simulink library "M160_lib"  (Simulink 7.8)
settings: Solver=FixedStepDiscrete  StartTime=0.0  StopTime=10.0  RelTol=1e-3
PreLoadFcn:
  | update_path
undefined symbols (not defined in the file): Afr_atCool2facLambdaReqCorr_CUR_x, Afr_atCool2facLambdaReqCorr_CUR_y, Afr_atMani2facLambdaReqCorr_CUR_x, Afr_atMani2facLambdaReqCorr_CUR_y, Afr_facLambdaReqMan, Afr_facRatioMan, Afr_facStoich, Afr_flgLambdaReqOverride, Afr_flgRatioOverride, Afr_rpmEngSpdfacRelAir2facLambdaReqBase_MAP_x, Afr_rpmEngSpdfacRelAir2facLambdaReqBase_MAP_y, Afr_rpmEngSpdfacRelAir2facLambdaReqBase_MAP_z, Ais_flgAirInjReacPumpOverride, Ais_stAirInjReacPumpMan, Amc_flgAirMassFlowOverride, Amc_uSens2AirMassFlow_CUR_x, Amc_uSens2AirMassFlow_CUR_y, Amc_uSensMaxValid, Amc_uSensMinValid, Amf_facRelAirMan, Amf_flgAirMassPerStrOverride, Amf_flgRelAirOverride, Amf_flgSwitch2AirMassFlowMeter, Amf_mAirPerStrMan, Amf_pManiEngSpd2facRelAirCorr_MAP_x, Amf_pManiEngSpd2facRelAirCorr_MAP_y, Amf_pManiEngSpd2facRelAirCorr_MAP_z, Amf_rpmEngSpd2facTempCorr_CUR_x, Amf_rpmEngSpd2facTempCorr_CUR_y, Amf_shcSpecGasConst_C, Amf_volEngDisp_C, Apv_facAirPumpRateMan, Apv_factor, Apv_flgAirPumpRateOverride, Apv_tiPeriod_C, Bvc_rVoltDivHigh, Bvc_rVoltDivLow, Bvc_uBattMax, Bvc_uBattMin, CDRV_E_OK_, Cov_facChOverVlvRateMan, Cov_factor, Cov_flgChOverVlvRateOverride, Cov_tiPeriod_C, Cpc_atManiTmp2facPresCorr_CUR_x, Cpc_atManiTmp2facPresCorr_CUR_y, Cpc_flgPChargeOverride, Cpc_uSens2pManiBase_CUR_x, Cpc_uSens2pManiBase_CUR_y, Ctc_rPullUp_C, Ctc_rSens2atCool_CUR_x, Ctc_rSens2atCool_CUR_y, Ctc_uSensMaxValid, Ctc_uSensMinValid, Ctc_uSupply, Doh_OutputDiagnosisOverride, dummy_facAirPumpRateReq, dummy_facChOverVlvRateReq, dummy_flgInterCoolerOverride, dummy_flgKl50Override ... (+243)
libraries: simulink x36, ehooks_lib x3
(part 8 of 8)

== system M160_lib/Sensors/Cpc/Cpc_get/G1_ADC_Input_Receive ==
  Data Type Conversion2 : DataTypeConversion  OutMin=0.0  OutMax=5.0  OutDataTypeStr=single
  Data Type Conversion3 : DataTypeConversion  OutMin=0.0  OutMax=1.0  OutDataTypeStr=boolean
  FlexECU_DevLib_FcnAPI_Wrapper_SFcn : S-Function  FunctionName=ehooks_medc17flex_devlib_basic_io_fcncall  Parameters=NoInputPorts, NoOutputPorts, InputPortDataTypes, OutputPortDataTypes, CFunctionArgTypes, CFunctionName, ChannelName  EnableBusSupport=off  mask{NoInputPorts=0, NoOutputPorts=2, InputPortDataTypes=, OutputPortDataTypes=uint8,int16, CFunctionArgTypes=ret,ref, CFunctionName=DevLib_Adc_Get, ChannelName=I_A_AN05}
      mask prompts: NoInputPorts "Number of input ports"; NoOutputPorts "Number of output ports"; InputPortDataTypes "Input port data types"; OutputPortDataTypes "Output port data types"; CFunctionArgTypes "C function argument types"; CFunctionName "C function name"; ChannelName "Channel (pin) name"
      mask Display: disp('EHOOKS FlexECU\nDevLib Wrapper\nS-Function')
  Gain : Gain  Gain=5/1023  OutDataTypeStr=Inherit: Same as input
  status : Outport
  uRaw : Outport  Port=2
  wires:
  FlexECU_DevLib_FcnAPI_Wrapper_SFcn/1 -> Data Type Conversion3/1
  FlexECU_DevLib_FcnAPI_Wrapper_SFcn/2 -> Data Type Conversion2/1
  Gain/1 -> uRaw/1
  Data Type Conversion3/1 -> status/1
  Data Type Conversion2/1 -> Gain/1

== system M160_lib/Sensors/Cpc/Cpc_pCharge_calc/ECU_FcnCallTrigger_Source_DownStream ==
  ECU_FcnCallTrigger_Source_SFcn : S-Function  Tag=ECU_FcnCallTrigger_Source_SFcn  Description=Internal S-function for custom block ECU_FcnCallTrigger_Source. Do not rename!  FunctionName=ehooks_fcncalltrigger_source  Parameters=FunctionBlockId, FunctionCName, ProcessName, TaskPeriod, TaskPriority  EnableBusSupport=off  mask(ECU_FcnCallTrigger_Source_SFcn){FunctionCName=Cpc_pCharge_calc, FunctionBlockId=SmartM160/Sensors/Cpc/Cpc_pCharge_calc, ProcessName=BypEasyhooks_S0_Pre_Proc, TaskPriority=0, TaskPeriod=1}
      mask prompts: FunctionCName "Function C name"; FunctionBlockId "Function block identifier"; ProcessName "Process name"; TaskPriority "Task priority (0..255)"; TaskPeriod "Sample time (0 for asynchronous operation)"
      mask help: Internal S-function for custom block ECU_FcnCallTrigger_Source. Do not rename!
      mask Display: disp('EHOOKS ECU Trigger\nSource S-Function')
  TriggerOut : Outport
  wires:
  ECU_FcnCallTrigger_Source_SFcn/1 -> TriggerOut/1

== system M160_lib/Sensors/Cpc/Cpc_pCharge_get/ECU_FcnCallTrigger_Source_DownStream ==
  ECU_FcnCallTrigger_Source_SFcn : S-Function  Tag=ECU_FcnCallTrigger_Source_SFcn  Description=Internal S-function for custom block ECU_FcnCallTrigger_Source. Do not rename!  FunctionName=ehooks_fcncalltrigger_source  Parameters=FunctionBlockId, FunctionCName, ProcessName, TaskPeriod, TaskPriority  EnableBusSupport=off  mask(ECU_FcnCallTrigger_Source_SFcn){FunctionCName=Cpc_pCharge_get, FunctionBlockId=SmartM160/Sensors/Cpc/Cpc_pCharge_get, ProcessName=BypEasyhooks_1ms_Pre_Proc, TaskPriority=0, TaskPeriod=1}
      mask prompts: FunctionCName "Function C name"; FunctionBlockId "Function block identifier"; ProcessName "Process name"; TaskPriority "Task priority (0..255)"; TaskPeriod "Sample time (0 for asynchronous operation)"
      mask help: Internal S-function for custom block ECU_FcnCallTrigger_Source. Do not rename!
      mask Display: disp('EHOOKS ECU Trigger\nSource S-Function')
  TriggerOut : Outport
  wires:
  ECU_FcnCallTrigger_Source_SFcn/1 -> TriggerOut/1

== system M160_lib/Sensors/Mpc/Mpc_calc/Accumulator ==
  in : Inport
  initValue : Inport  Port=2
  Add : Sum
  MATLAB Function : MATLAB Function  TreatAsAtomicUnit=on
  Switch2 : Switch  Threshold=1
  Unit Delay : UnitDelay  SampleTime=-1
  Out2 : Outport
  wires:
  MATLAB Function/1(y) -> Switch2/2
  Add/1 -> Unit Delay/1, Switch2/1
  initValue/1 -> Switch2/3
  Switch2/1 -> Out2/1
  Unit Delay/1 -> Add/2
  in/1 -> MATLAB Function/1(u), Add/1

== system M160_lib/Sensors/Mpc/Mpc_calc/Counter ==
  in : Inport
  Add1 : Sum
  Constant1 : Constant  OutDataTypeStr=single
  Constant2 : Constant  Value=0  OutDataTypeStr=single
  MATLAB Function : MATLAB Function  TreatAsAtomicUnit=on
  Switch2 : Switch  Threshold=1
  Unit Delay1 : UnitDelay  SampleTime=-1
  Out1 : Outport
  wires:
  in/1 -> MATLAB Function/1(u)
  MATLAB Function/1(y) -> Switch2/2
  Add1/1 -> Unit Delay1/1, Switch2/1
  Constant2/1 -> Switch2/3
  Switch2/1 -> Out1/1
  Unit Delay1/1 -> Add1/2
  Constant1/1 -> Add1/1

== system M160_lib/Sensors/Mpc/Mpc_get/G1_ADC_Input_Receive ==
  Data Type Conversion2 : DataTypeConversion  OutMin=0.0  OutMax=5.0  OutDataTypeStr=single
  Data Type Conversion3 : DataTypeConversion  OutMin=0.0  OutMax=1.0  OutDataTypeStr=boolean
  FlexECU_DevLib_FcnAPI_Wrapper_SFcn : S-Function  FunctionName=ehooks_medc17flex_devlib_basic_io_fcncall  Parameters=NoInputPorts, NoOutputPorts, InputPortDataTypes, OutputPortDataTypes, CFunctionArgTypes, CFunctionName, ChannelName  EnableBusSupport=off  mask{NoInputPorts=0, NoOutputPorts=2, InputPortDataTypes=, OutputPortDataTypes=uint8,int16, CFunctionArgTypes=ret,ref, CFunctionName=DevLib_Adc_Get, ChannelName=I_A_AN05}
      mask prompts: NoInputPorts "Number of input ports"; NoOutputPorts "Number of output ports"; InputPortDataTypes "Input port data types"; OutputPortDataTypes "Output port data types"; CFunctionArgTypes "C function argument types"; CFunctionName "C function name"; ChannelName "Channel (pin) name"
      mask Display: disp('EHOOKS FlexECU\nDevLib Wrapper\nS-Function')
  Gain : Gain  Gain=5/1023  OutDataTypeStr=Inherit: Same as input
  status : Outport
  uRaw : Outport  Port=2
  wires:
  Data Type Conversion2/1 -> Gain/1
  Data Type Conversion3/1 -> status/1
  Gain/1 -> uRaw/1
  FlexECU_DevLib_FcnAPI_Wrapper_SFcn/2 -> Data Type Conversion2/1
  FlexECU_DevLib_FcnAPI_Wrapper_SFcn/1 -> Data Type Conversion3/1

== system M160_lib/Sensors/Mpc/Mpc_pMani_calc/ECU_FcnCallTrigger_Source_DownStream ==
  ECU_FcnCallTrigger_Source_SFcn : S-Function  Tag=ECU_FcnCallTrigger_Source_SFcn  Description=Internal S-function for custom block ECU_FcnCallTrigger_Source. Do not rename!  FunctionName=ehooks_fcncalltrigger_source  Parameters=FunctionBlockId, FunctionCName, ProcessName, TaskPeriod, TaskPriority  EnableBusSupport=off  mask(ECU_FcnCallTrigger_Source_SFcn){FunctionCName=Mpc_pMani_calc, FunctionBlockId=SmartM160/Sensors/Mpc/Mpc_pMani_calc, ProcessName=BypEasyhooks_S0_Pre_Proc, TaskPriority=0, TaskPeriod=1}
      mask prompts: FunctionCName "Function C name"; FunctionBlockId "Function block identifier"; ProcessName "Process name"; TaskPriority "Task priority (0..255)"; TaskPeriod "Sample time (0 for asynchronous operation)"
      mask help: Internal S-function for custom block ECU_FcnCallTrigger_Source. Do not rename!
      mask Display: disp('EHOOKS ECU Trigger\nSource S-Function')
  TriggerOut : Outport
  wires:
  ECU_FcnCallTrigger_Source_SFcn/1 -> TriggerOut/1

== system M160_lib/Sensors/Mpc/Mpc_pMani_get/ECU_FcnCallTrigger_Source_DownStream ==
  ECU_FcnCallTrigger_Source_SFcn : S-Function  Tag=ECU_FcnCallTrigger_Source_SFcn  Description=Internal S-function for custom block ECU_FcnCallTrigger_Source. Do not rename!  FunctionName=ehooks_fcncalltrigger_source  Parameters=FunctionBlockId, FunctionCName, ProcessName, TaskPeriod, TaskPriority  EnableBusSupport=off  mask(ECU_FcnCallTrigger_Source_SFcn){FunctionCName=Mpc_pMani_get, FunctionBlockId=SmartM160/Sensors/Mpc/Mpc_pMani_get, ProcessName=BypEasyhooks_1ms_Pre_Proc, TaskPriority=0, TaskPeriod=1}
      mask prompts: FunctionCName "Function C name"; FunctionBlockId "Function block identifier"; ProcessName "Process name"; TaskPriority "Task priority (0..255)"; TaskPeriod "Sample time (0 for asynchronous operation)"
      mask help: Internal S-function for custom block ECU_FcnCallTrigger_Source. Do not rename!
      mask Display: disp('EHOOKS ECU Trigger\nSource S-Function')
  TriggerOut : Outport
  wires:
  ECU_FcnCallTrigger_Source_SFcn/1 -> TriggerOut/1

== system M160_lib/Actuators/Tvc/ThrottleValveControl/PID_Limit_AWU/Limiter ==
  max : Inport
  in : Inport  Port=2
  min : Inport  Port=3
  Saturation Dynamic : simulink/Discontinuities/Saturation Dynamic  OutMin=[]  OutMax=[]  OutDataTypeStr=Inherit: Same as second input  OutDataType=fixdt(1, 16)  OutScaling=2^-10  DoSatur=off
  return : Outport
  wires:
  max/1 -> Saturation Dynamic/1
  in/1 -> Saturation Dynamic/2
  min/1 -> Saturation Dynamic/3
  Saturation Dynamic/1 -> return/1

== system M160_lib/Functions/Lcc/PID-Controller/PID_Limit_AWU/Limiter ==
  max : Inport
  in : Inport  Port=2
  min : Inport  Port=3
  Saturation Dynamic : simulink/Discontinuities/Saturation Dynamic  OutMin=[]  OutMax=[]  OutDataTypeStr=Inherit: Same as second input  OutDataType=fixdt(1, 16)  OutScaling=2^-10  DoSatur=off
  return : Outport
  wires:
  max/1 -> Saturation Dynamic/1
  in/1 -> Saturation Dynamic/2
  min/1 -> Saturation Dynamic/3
  Saturation Dynamic/1 -> return/1

== system M160_lib/Functions/T2t/ThrottleValveControl/PID_Limit_AWU/Limiter ==
  max : Inport
  in : Inport  Port=2
  min : Inport  Port=3
  Saturation Dynamic : simulink/Discontinuities/Saturation Dynamic  OutMin=[]  OutMax=[]  OutDataTypeStr=Inherit: Same as second input  OutDataType=fixdt(1, 16)  OutScaling=2^-10  DoSatur=off
  return : Outport
  wires:
  max/1 -> Saturation Dynamic/1
  in/1 -> Saturation Dynamic/2
  min/1 -> Saturation Dynamic/3
  Saturation Dynamic/1 -> return/1

== system M160_lib/Functions/T2t/WastegateControl/PID_Limit_AWU/Limiter ==
  max : Inport
  in : Inport  Port=2
  min : Inport  Port=3
  Saturation Dynamic : simulink/Discontinuities/Saturation Dynamic  OutMin=[]  OutMax=[]  OutDataTypeStr=Inherit: Same as second input  OutDataType=fixdt(1, 16)  OutScaling=2^-10  DoSatur=off
  return : Outport
  wires:
  Saturation Dynamic/1 -> return/1
  min/1 -> Saturation Dynamic/3
  in/1 -> Saturation Dynamic/2
  max/1 -> Saturation Dynamic/1

== system M160_lib/Functions/Tqs/EngSpdControl/PID_Limit_AWU/Limiter ==
  max : Inport
  in : Inport  Port=2
  min : Inport  Port=3
  Saturation Dynamic : simulink/Discontinuities/Saturation Dynamic  OutMin=[]  OutMax=[]  OutDataTypeStr=Inherit: Same as second input  OutDataType=fixdt(1, 16)  OutScaling=2^-10  DoSatur=off
  return : Outport
  wires:
  max/1 -> Saturation Dynamic/1
  in/1 -> Saturation Dynamic/2
  min/1 -> Saturation Dynamic/3
  Saturation Dynamic/1 -> return/1

== matlab function Sensors/Egc/LowpassT/MATLAB Function ==
  data: x output double; u input double; y output double
function [x,y]= fcn(u)
% initValue Test
if(u<0)
    y = 0;
else
    y = 1;
end

x = u;

== matlab function Sensors/Egc/LowpassT_Fcn/MATLAB Function ==
  data: u input double; y output double
function y = fcn(u)
% initValue Test
if(u<0)
    y = 0;
else
    y = 1;
end

== matlab function Sensors/Cpc/Cpc_calc/Accumulator/MATLAB Function ==
  data: u input double; y output double
function y = fcn(u)
% initValue Test
if(u<=0)
    y = 0;
else
    y = 1;
end

== matlab function Sensors/Cpc/Cpc_calc/Counter/MATLAB Function ==
  data: u input double; y output double
function y = fcn(u)
% initValue Test
if(u<=0)
    y = 0;
else
    y = 1;
end

== matlab function Functions/Opm/OpMode/fcn_OpMode ==
  data: Opm_stEngControl input double; Opm_flgIOErrorAct input double; Opm_idxAct output double; Opm_flgIOErrorMemIn input double; Opm_flgIOErrorReset output double
function [Opm_idxAct,Opm_flgIOErrorReset]= fcn(Opm_stEngControl,Opm_flgIOErrorAct,Opm_flgIOErrorMemIn)
% fcn_OpMode

sm = single(0);
Opm_idxAct = single(0);
Opm_flgIOErrorReset = false;

if(sm==0)                                            % Off_state
        if(Opm_stEngControl)
            Opm_idxAct = single(1);
            sm = single(2);
        end
        if(Opm_flgIOErrorMemIn)
            Opm_idxAct = single(2);
            sm = single(1);
        end
        Opm_flgIOErrorReset = false;
end
if(sm==1)                                            % IOError_state
        if((~Opm_stEngControl)&&(~Opm_flgIOErrorAct))
            Opm_flgIOErrorReset = true;
            Opm_idxAct = single(0);
            sm = single(0);
        end
end
if(sm==2)                                            % Normal_state
        if(~Opm_stEngControl)
            Opm_idxAct = single(0);
            sm = single(0);
        end
        if(Opm_flgIOErrorMemIn)
            Opm_idxAct = single(2);
            sm = single(1);
        end
        Opm_flgIOErrorReset = false;
end

== matlab function Functions/Opm/ErrorCheck/Counter/MATLAB Function ==
  data: u input double; y output double
function y = fcn(u)
% initValue Test
if(u<=0)
    y = 0;
else
    y = 1;
end

== matlab function Functions/Opm/ErrorCheck/Counter1/MATLAB Function ==
  data: u input double; y output double
function y = fcn(u)
% initValue Test
if(u<=0)
    y = 0;
else
    y = 1;
end

== matlab function Functions/Opm/ErrorCheck/Counter2/MATLAB Function ==
  data: u input double; y output double
function y = fcn(u)
% initValue Test
if(u<=0)
    y = 0;
else
    y = 1;
end

== matlab function Sensors/Mpc/Mpc_calc/Accumulator/MATLAB Function ==
  data: u input double; y output double
function y = fcn(u)
% initValue Test
if(u<=0)
    y = 0;
else
    y = 1;
end

== matlab function Sensors/Mpc/Mpc_calc/Counter/MATLAB Function ==
  data: u input double; y output double
function y = fcn(u)
% initValue Test
if(u<=0)
    y = 0;
else
    y = 1;
end

== matlab function Functions/ICC_1/RSFlipFlop/MATLAB Function ==
  data: r input double; q output double; s input double
function q = fcn(r,s)
% FlipFlop
q = false;
if(r==true)
    q = false;
elseif(s==true)
    q = true;
end

== matlab function Functions/Stc/RSFlipFlop/MATLAB Function ==
  data: r input double; q output double; s input double
function q = fcn(r,s)
% FlipFlop
q = false;
if(r==true)
    q = false;
elseif(s==true)
    q = true;
end

== matlab function Functions/Stc/CounterEnabled/MATLAB Function ==
  data: u input double; y output double; v input double
function y = fcn(u,v)
% CounterEnabled Test
y = false;
if(u==true)
    y = false;
end
if(v==true)
    y = true;
end

== matlab function Functions/Stc/RSFlipFlop1/MATLAB Function ==
  data: r input double; q output double; s input double
function q = fcn(r,s)
% FlipFlop
q = false;
if(r==true)
    q = false;
elseif(s==true)
    q = true;
end

== matlab function Functions/Stc/RSFlipFlop2/MATLAB Function ==
  data: r input double; q output double; s input double
function q = fcn(r,s)
% FlipFlop
q = false;
if(r==true)
    q = false;
elseif(s==true)
    q = true;
end

== matlab function Functions/Stc/RSFlipFlop3/MATLAB Function ==
  data: r input double; q output double; s input double
function q = fcn(r,s)
% FlipFlop
q = false;
if(r==true)
    q = false;
elseif(s==true)
    q = true;
end

== matlab function Functions/Stc/CounterEnabled1/MATLAB Function ==
  data: u input double; y output double; v input double
function y = fcn(u,v)
% CounterEnabled Test
y = false;
if(u==true)
    y = false;
end
if(v==true)
    y = true;
end

== matlab function Functions/Lcc/Two-point-controller/Integrator/MATLAB Function ==
  data: initEnable input double; out output double; initValue input double; enable input double; in input double
function out = fcn(initEnable,initValue,enable,in)
% Integrator Test
out = single(0.0);
if(initEnable==true)
    out = initValue;
end
if(enable==true)
    out = single(in);
end

== matlab function Functions/Isc/Integrator/MATLAB Function ==
  data: initEnable input double; out output double; initValue input double; enable input double; in input double
function out = fcn(initEnable,initValue,enable,in)
% Integrator Test
out = single(0.0);
if(initEnable==true)
    out = initValue;
end
if(enable==true)
    out = single(in);
end

== matlab function Functions/Isc/CounterEnabled/MATLAB Function ==
  data: u input double; y output double; v input double
function y = fcn(u,v)
% CounterEnabled Test
y = false;
if(u==true)
    y = false;
end
if(v==true)
    y = true;
end

== matlab function Functions/Isc/Integrator1/MATLAB Function ==
  data: initEnable input double; out output double; initValue input double; enable input double; in input double
function out = fcn(initEnable,initValue,enable,in)
% Integrator Test
out = single(0.0);
if(initEnable==true)
    out = initValue;
end
if(enable==true)
    out = single(in);
end
